simulink model "sistema_motor_planta_aproximacao_restored_from_autosave"  (R2024b)
settings: Solver=VariableStepAuto  StartTime=0.0  StopTime=10.0  RelTol=1e-3
settings Model: Creator=kayky  LastModifiedBy=kayky.jesus

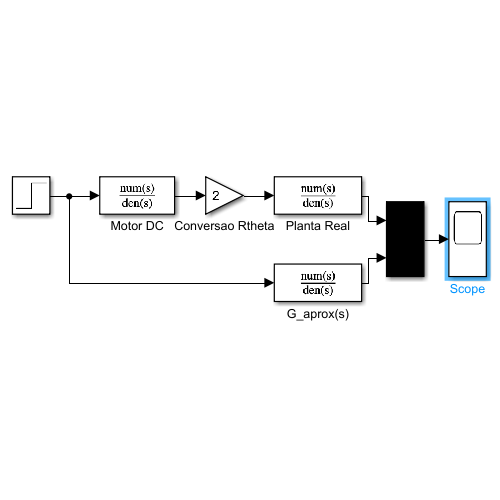
[thumbnail: Simulink's stored preview of the top-level diagram]
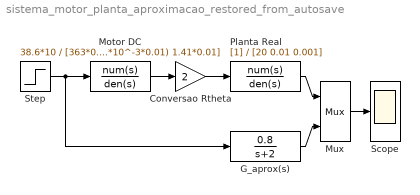
== system sistema_motor_planta_aproximacao_restored_from_autosave ==
  Conversao Rtheta : Gain  Gain=2
  G_aprox(s) : TransferFcn  Numerator=0.8  Denominator=[1 2]
  Motor DC : TransferFcn  Numerator=38.6*10  Denominator=[363*0.281*10^-3 (363*1.41 + 0.281*10^-3*0.01) 1.41*0.01]
  Mux : Mux  Inputs=2
  Planta Real : TransferFcn  Denominator=[20 0.01 0.001]
  Scope : Scope
  Step : Step  Time=0  SampleTime=0
  wires:
  Step/1 -> G_aprox(s)/1, Motor DC/1
  Motor DC/1 -> Conversao Rtheta/1
  Conversao Rtheta/1 -> Planta Real/1
  Planta Real/1 -> Mux/1
  G_aprox(s)/1 -> Mux/2
  Mux/1 -> Scope/1
